simulink model "MPC_Pseudostatess_with_psif"  (R2020a)
settings: Solver=VariableStepAuto  StartTime=0.0  StopTime=10.0  RelTol=1e-3
values from neighbouring files (symbols this model uses):
  kp = 0.001    [init.m]    (also in matlab.mat)
  l = 0.25    [init.m]    (also in matlab.mat)
libraries: mpclib x1, cstblocks x1

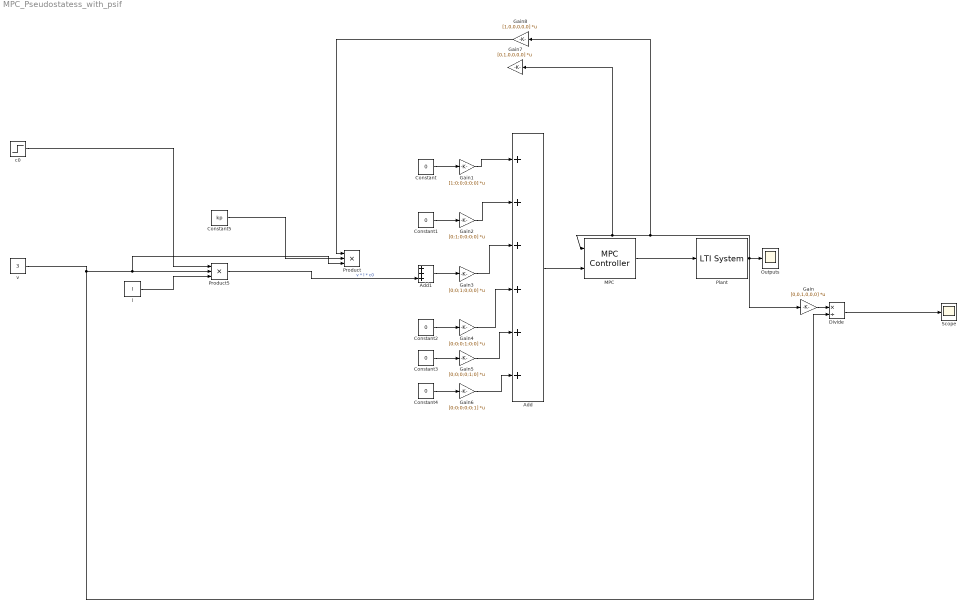
== system MPC_Pseudostatess_with_psif ==
  Add : Sum  Inputs=++++++
  Add1 : Sum  Inputs=+++
  Constant{,1..4} (5 alike) : Constant  Value=0
  Constant5 : Constant  Value=kp
  Divide : Product  Inputs=*/
  Gain : Gain  Gain=[0,0,1,0,0,0]  Multiplication=Matrix(K*u)
  Gain1 : Gain  Gain=[1;0;0;0;0;0]  Multiplication=Matrix(K*u)
  Gain2 : Gain  Gain=[0;1;0;0;0;0]  Multiplication=Matrix(K*u)
  Gain3 : Gain  Gain=[0;0;1;0;0;0]  Multiplication=Matrix(K*u)
  Gain4 : Gain  Gain=[0;0;0;1;0;0]  Multiplication=Matrix(K*u)
  Gain5 : Gain  Gain=[0;0;0;0;1;0]  Multiplication=Matrix(K*u)
  Gain6 : Gain  Gain=[0;0;0;0;0;1]  Multiplication=Matrix(K*u)
  Gain7 : Gain  Gain=[0,1,0,0,0,0]  Multiplication=Matrix(K*u)
  Gain8 : Gain  Gain=[1,0,0,0,0,0]  Multiplication=Matrix(K*u)
  MPC : mpclib/MPC Controller  SCDEnableBlockLinearizationSpecification=on  mpcobj=mpc1_1_C_4  is_multiple=0  enable_value=0  return_u0=off  updateMPCinCallerWorkspace=on  md_inport=off  mv_inport=off  uref_inport=off  return_cost=off  return_mvseq=off  return_qpstatus=off  return_xseq=off  return_state=off  return_ovseq=off  state_inport=off  umin_inport=off  umax_inport=off  ymin_inport=off  ymax_inport=off  cc_inport=off  ywt_inport=off  uwt_inport=off  duwt_inport=off  rhoeps_inport=off  pm_inport=off  MaximumP=10  HorizonChoice=FixedHorizon  n_ts=0.05  n_p=10  n_mv=5  n_md=0  n_ud=0  n_mo=6  n_uo=0  BlockDataType=double  SampleTimeInherited=off  switch_inport=off
  Outputs : Scope
  Plant : cstblocks/LTI System  sys=mpc1_1_G_4  IC=[]
  Product : Product  Inputs=3
  Product5 : Product  Inputs=3
  Scope : Scope
  c0 : Step  SampleTime=0
  l : Constant  Value=l
  v : Constant  Value=3
  wires:
  Plant/1 -> Gain8/1, Gain7/1, MPC/1, Gain/1, Outputs/1
  MPC/1 -> Plant/1
  Divide/1 -> Scope/1
  v/1 -> Product/3, Product5/2, Divide/2
  Gain/1 -> Divide/1
  Constant/1 -> Gain1/1
  Constant1/1 -> Gain2/1
  Constant2/1 -> Gain4/1
  c0/1 -> Product5/1
  Gain2/1 -> Add/2
  Gain3/1 -> Add/3
  Gain4/1 -> Add/4
  l/1 -> Product5/3
  Add/1 -> MPC/2
  Gain1/1 -> Add/1
  Gain5/1 -> Add/5
  Constant3/1 -> Gain5/1
  Gain6/1 -> Add/6
  Constant4/1 -> Gain6/1
  Add1/1 -> Gain3/1
  Product5/1 -> Add1/3  "v * l * c0"
  Gain8/1 -> Product/1
  Constant5/1 -> Product/2
